simulink model "three_phase_pwm_rectifier_with_PMSGblock"  (R2015b)
settings: Solver=FixedStepAuto  SolverMode=SingleTasking  StartTime=0.0  StopTime=10.0  FixedStep=Ts  RelTol=1e-3
values from neighbouring files (symbols this model uses):
  Ts = 10e-6    (= 1e-05)    [three_phase_pwm_rectifier.m]
undefined symbols (not defined in the file or in its folder): fluxlinkage, gear, Jtotal, Ld, Lq, p, pgen, Prated, R, Rs, windspeed
libraries: powerlib x23, powerlib_meascontrol x9, simulink x7
settings Model: Creator=Eren  LastModifiedBy=Eren

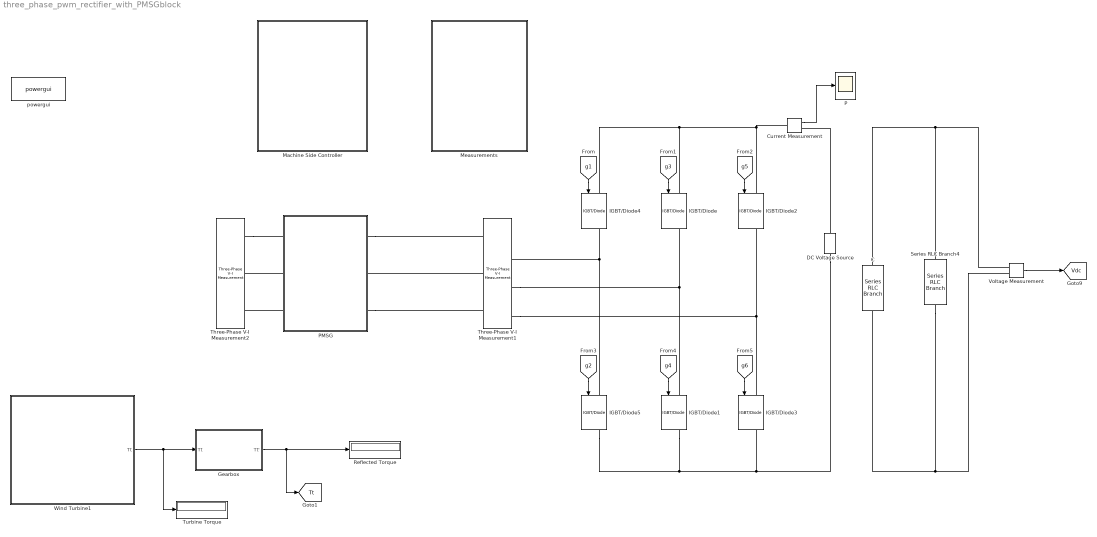
== system three_phase_pwm_rectifier_with_PMSGblock ==
  C : powerlib/Elements/Series RLC Branch  LConnTagsString=__new0  RConnTagsString=__new0  BranchType=C  Resistance=1  Inductance=1e-3  SetiL0=off  InitialCurrent=0  Capacitance=2700e-6  Setx0=on  InitialVoltage=1200  Measurements=None
  Current Measurement : powerlib/Measurements/Current Measurement  PhasorSimulation=off  OutputType=Complex  PSBequivalent=0
  DC Voltage Source : powerlib/Electrical Sources/DC Voltage Source  Amplitude=1200  Measurements=None
  Gearbox : Subsystem
  IGBT/Diode{,1..5} (6 alike) : powerlib/Power Electronics/IGBT//Diode  Ron=1e-3  Rs=1e5  Cs=inf  Measurements=on
  "Machine Side Controller " : Subsystem
  Measurements : Subsystem
  P : Scope
  "PMSG " : Subsystem
  Reflected Torque : Display
  Series RLC Branch4 : powerlib/Elements/Series RLC Branch  LConnTagsString=__new0  RConnTagsString=__new0  BranchType=R  Resistance=(1200)^2/2.75e6  Inductance=1e-3  SetiL0=off  InitialCurrent=0  Capacitance=1e-6  Setx0=off  InitialVoltage=0  Measurements=None
  Three-Phase V-I Measurement1 : powerlib/Measurements/Three-Phase V-I Measurement  VoltageMeasurement=phase-to-phase  SetLabelV=off  LabelV=Vsabc  Vpu=off  VpuLL=on  CurrentMeasurement=yes  SetLabelI=on  LabelI=Isabc  Ipu=on  Pbase=2.75e6  Vbase=690  OutputType=Complex  PhasorSimulation=off  PSBequivalent=0
  Three-Phase V-I Measurement2 : powerlib/Measurements/Three-Phase V-I Measurement  VoltageMeasurement=phase-to-phase  SetLabelV=on  LabelV=Vsabc  Vpu=off  VpuLL=on  CurrentMeasurement=no  SetLabelI=off  LabelI=Isabc  Ipu=off  Pbase=2.75e6  Vbase=690  OutputType=Complex  PhasorSimulation=off  PSBequivalent=0
  Turbine Torque : Display
  Voltage Measurement : powerlib/Measurements/Voltage Measurement  PhasorSimulation=off  OutputType=Complex  PSBequivalent=0
  Wind Turbine1 : Subsystem
  powergui : powerlib/powergui  Priority=2  SimulationMode=Discrete  SolverType=Tustin  SampleTime=Ts  frequency=60  SPID=off  DisableSnubberDevices=off  DisableRonSwitches=off  DisableVfSwitches=off  SwTol=0  DisplayEquations=off  Interpol=off  ExternalGateDelay=off  methode=off  Ts=0  FunctionMessages=off  echomessages=off  HookPort=off  EnableUseOfTLC=off  x0status=blocks  frequencyindice=0  Pbase=100e6  ErrMax=1e-4  Iterations=50  UnitsV=kV  UnitsW=MW  buscounter=0  RestoreLinks=warning  ResistiveCurrentMeasurement=off  Frange=[0:2:500]  Ylog=off  Xlog=on  ShowGrid=off  save=off  variable=ZData  structure=0  ZoomFFT=on  StartTime=0.0  cycles=1  DisplayStyle=1  fundamental=60  FreqAxis=off  MaxFrequency=1000  frequencyindicesteady=1  RmsSteady=1  display=off
  tag scope: Tt=global, Vdc=global
  wires:
  [g1] -> IGBT/Diode4/1
  [g3] -> IGBT/Diode/1
  [g5] -> IGBT/Diode2/1
  [g2] -> IGBT/Diode5/1
  [g4] -> IGBT/Diode1/1
  [g6] -> IGBT/Diode3/1
  Voltage Measurement/1 -> [Vdc]
  Current Measurement/1 -> P/1
  Wind Turbine1/1(Tt) -> Turbine Torque/1, Gearbox/1(Tt)
  Gearbox/1(Tt') -> [Tt], Reflected Torque/1
  connections:
  IGBT/Diode5/LConn1 -- IGBT/Diode4/RConn1 -- Three-Phase V-I Measurement1/RConn1
  IGBT/Diode1/LConn1 -- Three-Phase V-I Measurement1/RConn2 -- IGBT/Diode/RConn1
  IGBT/Diode3/LConn1 -- Three-Phase V-I Measurement1/RConn3 -- IGBT/Diode2/RConn1
  Series RLC Branch4/LConn1 -- Voltage Measurement/LConn1 -- C/LConn1
  IGBT/Diode2/LConn1 -- Current Measurement/LConn1 -- IGBT/Diode/LConn1 -- IGBT/Diode4/LConn1
  Voltage Measurement/LConn2 -- C/RConn1 -- Series RLC Branch4/RConn1
  "PMSG "/RConn1 -- Three-Phase V-I Measurement1/LConn1
  IGBT/Diode5/RConn1 -- IGBT/Diode3/RConn1 -- DC Voltage Source/LConn1 -- IGBT/Diode1/RConn1
  DC Voltage Source/RConn1 -- Current Measurement/RConn1
  "PMSG "/RConn3 -- Three-Phase V-I Measurement1/LConn3
  Three-Phase V-I Measurement1/LConn2 -- "PMSG "/RConn2
  Three-Phase V-I Measurement2/RConn1 -- "PMSG "/LConn1
  "PMSG "/LConn2 -- Three-Phase V-I Measurement2/RConn2
  "PMSG "/LConn3 -- Three-Phase V-I Measurement2/RConn3

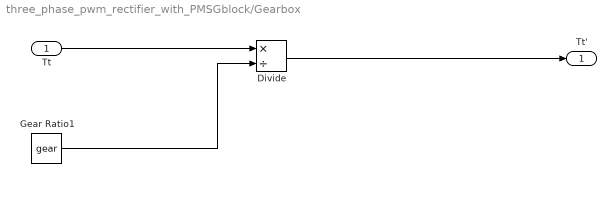
== system three_phase_pwm_rectifier_with_PMSGblock/Gearbox ==
  Tt : Inport
  Divide : Product  Inputs=*/
  Gear Ratio1 : Constant  Value=gear
  Tt' : Outport
  wires:
  Gear Ratio1/1 -> Divide/2
  Tt/1 -> Divide/1
  Divide/1 -> Tt'/1

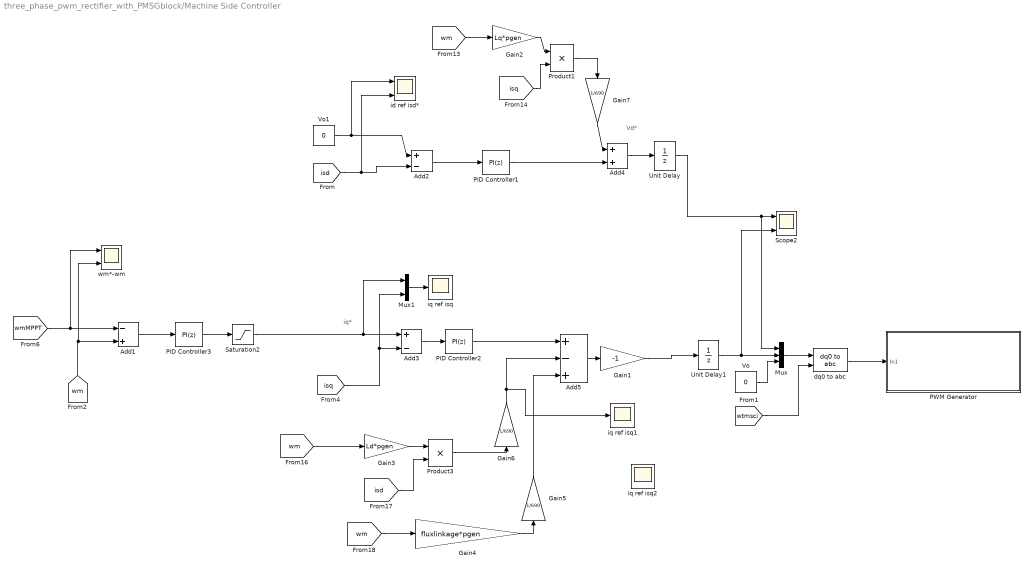
== system three_phase_pwm_rectifier_with_PMSGblock/Machine Side Controller  ==
  note: iq*
  note: Vd*
  Add1 : Sum  Inputs=-+
  Add2 : Sum  Inputs=+-
  Add3 : Sum  Inputs=+-
  Add4 : Sum
  Add5 : Sum  Inputs=+-+
  Gain1 : Gain  Gain=-1
  Gain2 : Gain  Gain=Lq*pgen
  Gain3 : Gain  Gain=Ld*pgen
  Gain4 : Gain  Gain=fluxlinkage*pgen
  Gain5 : Gain  Gain=1/690
  Gain6 : Gain  Gain=1/690
  Gain7 : Gain  Gain=1/690
  Mux : Mux  Inputs=3
  Mux1 : Mux  Inputs=2
  PID Controller1 : simulink/Continuous/PID Controller  Controller=PI  TimeDomain=Discrete-time  SampleTime=-1  IntegratorMethod=Forward Euler  FilterMethod=Forward Euler  Form=Ideal  UseFilter=on  ControllerParametersSource=internal  P=0.01  I=0.1  D=0  N=100  InitialConditionSource=internal  InitialConditionForIntegrator=0  InitialConditionForFilter=0  ExternalReset=none  LimitOutput=on  UpperSaturationLimit=1.5  LowerSaturationLimit=-1.5  LinearizeAsGain=on  AntiWindupMode=none  Kb=1  TrackingMode=off  Kt=1  PParamMin=[]  PParamMax=[]  IParamMin=[]  IParamMax=[]  DParamMin=[]  DParamMax=[]  NParamMin=[]  NParamMax=[]  KbParamMin=[]  KbParamMax=[]  KtParamMin=[]  KtParamMax=[]  POutMin=[]  POutMax=[]  IOutMin=[]  IOutMax=[]  DOutMin=[]  DOutMax=[]  NOutMin=[]  NOutMax=[]  KbOutMin=[]  KbOutMax=[]  KtOutMin=[]  KtOutMax=[]  IntegratorOutMin=[]  IntegratorOutMax=[]  FilterOutMin=[]  FilterOutMax=[]  SumOutMin=[]  SumOutMax=[]  SumI1OutMin=[]  SumI1OutMax=[]  SumI2OutMin=[]  SumI2OutMax=[]  SumI3OutMin=[]  SumI3OutMax=[]  SumDOutMin=[]  SumDOutMax=[]  SaturationOutMin=[]  SaturationOutMax=[]  IntegratorContinuousStateAttributes=''  IntegratorStateMustResolveToSignalObject=off  IntegratorRTWStateStorageClass=Auto  FilterContinuousStateAttributes=''  FilterStateMustResolveToSignalObject=off  FilterRTWStateStorageClass=Auto  DifferentiatorICPrevScaledInput=0  DifferentiatorOutMin=[]  DifferentiatorOutMax=[]
  PID Controller2 : simulink/Continuous/PID Controller  Controller=PI  TimeDomain=Discrete-time  SampleTime=-1  IntegratorMethod=Forward Euler  FilterMethod=Forward Euler  Form=Ideal  UseFilter=on  ControllerParametersSource=internal  P=0.1  I=1  D=0  N=100  InitialConditionSource=internal  InitialConditionForIntegrator=0  InitialConditionForFilter=0  ExternalReset=none  LimitOutput=on  UpperSaturationLimit=1.5  LowerSaturationLimit=-1.5  LinearizeAsGain=on  AntiWindupMode=none  Kb=1  TrackingMode=off  Kt=1  PParamMin=[]  PParamMax=[]  IParamMin=[]  IParamMax=[]  DParamMin=[]  DParamMax=[]  NParamMin=[]  NParamMax=[]  KbParamMin=[]  KbParamMax=[]  KtParamMin=[]  KtParamMax=[]  POutMin=[]  POutMax=[]  IOutMin=[]  IOutMax=[]  DOutMin=[]  DOutMax=[]  NOutMin=[]  NOutMax=[]  KbOutMin=[]  KbOutMax=[]  KtOutMin=[]  KtOutMax=[]  IntegratorOutMin=[]  IntegratorOutMax=[]  FilterOutMin=[]  FilterOutMax=[]  SumOutMin=[]  SumOutMax=[]  SumI1OutMin=[]  SumI1OutMax=[]  SumI2OutMin=[]  SumI2OutMax=[]  SumI3OutMin=[]  SumI3OutMax=[]  SumDOutMin=[]  SumDOutMax=[]  SaturationOutMin=[]  SaturationOutMax=[]  IntegratorContinuousStateAttributes=''  IntegratorStateMustResolveToSignalObject=off  IntegratorRTWStateStorageClass=Auto  FilterContinuousStateAttributes=''  FilterStateMustResolveToSignalObject=off  FilterRTWStateStorageClass=Auto  DifferentiatorICPrevScaledInput=0  DifferentiatorOutMin=[]  DifferentiatorOutMax=[]
  PID Controller3 : simulink/Continuous/PID Controller  Controller=PI  TimeDomain=Discrete-time  SampleTime=-1  IntegratorMethod=Forward Euler  FilterMethod=Forward Euler  Form=Ideal  UseFilter=on  ControllerParametersSource=internal  P=0.01  I=0.001  D=0  N=100  InitialConditionSource=internal  InitialConditionForIntegrator=0  InitialConditionForFilter=0  ExternalReset=none  LimitOutput=on  UpperSaturationLimit=1.5  LowerSaturationLimit=-1.5  LinearizeAsGain=on  AntiWindupMode=none  Kb=1  TrackingMode=off  Kt=1  PParamMin=[]  PParamMax=[]  IParamMin=[]  IParamMax=[]  DParamMin=[]  DParamMax=[]  NParamMin=[]  NParamMax=[]  KbParamMin=[]  KbParamMax=[]  KtParamMin=[]  KtParamMax=[]  POutMin=[]  POutMax=[]  IOutMin=[]  IOutMax=[]  DOutMin=[]  DOutMax=[]  NOutMin=[]  NOutMax=[]  KbOutMin=[]  KbOutMax=[]  KtOutMin=[]  KtOutMax=[]  IntegratorOutMin=[]  IntegratorOutMax=[]  FilterOutMin=[]  FilterOutMax=[]  SumOutMin=[]  SumOutMax=[]  SumI1OutMin=[]  SumI1OutMax=[]  SumI2OutMin=[]  SumI2OutMax=[]  SumI3OutMin=[]  SumI3OutMax=[]  SumDOutMin=[]  SumDOutMax=[]  SaturationOutMin=[]  SaturationOutMax=[]  IntegratorContinuousStateAttributes=''  IntegratorStateMustResolveToSignalObject=off  IntegratorRTWStateStorageClass=Auto  FilterContinuousStateAttributes=''  FilterStateMustResolveToSignalObject=off  FilterRTWStateStorageClass=Auto  DifferentiatorICPrevScaledInput=0  DifferentiatorOutMin=[]  DifferentiatorOutMax=[]
  "PWM Generator " : Subsystem
  Product1 : Product
  Product3 : Product
  Saturation2 : Saturate  UpperLimit=1.5  LowerLimit=0
  Scope2 : Scope  NumInputPorts=2
  Unit Delay : UnitDelay  SampleTime=Ts
  Unit Delay1 : UnitDelay  SampleTime=Ts
  Vo : Constant  Value=0
  Vo1 : Constant  Value=0
  dq0 to abc : powerlib_meascontrol/Transformations/dq0 to abc  Alignment=Aligned with phase A axis
  id ref isd* : Scope  NumInputPorts=2
  iq ref isq : Scope
  iq ref isq1 : Scope
  iq ref isq2 : Scope
  wm*-wm : Scope  NumInputPorts=2
  wires:
  Mux/1 -> dq0 to abc/1
  Vo1/1 -> id ref isd*/1, Add2/1
  Vo/1 -> Mux/3
  [isq] -> Add3/2, Mux1/2
  Add3/1 -> PID Controller2/1
  Add2/1 -> PID Controller1/1
  [isd] -> id ref isd*/2, Add2/2
  Mux1/1 -> iq ref isq/1
  [wtmsci] -> dq0 to abc/2
  [wm] -> wm*-wm/2, Add1/2
  [wmMPPT] -> wm*-wm/1, Add1/1
  Add1/1 -> PID Controller3/1
  dq0 to abc/1 -> "PWM Generator "/1(In1)
  Unit Delay/1 -> Mux/1, Scope2/1
  Unit Delay1/1 -> Mux/2, Scope2/2
  [wm] -> Gain2/1
  [isq] -> Product1/2
  Gain2/1 -> Product1/1
  Add4/1 -> Unit Delay/1
  PID Controller1/1 -> Add4/2
  Add5/1 -> Gain1/1
  PID Controller2/1 -> Add5/1
  [wm] -> Gain3/1
  Gain3/1 -> Product3/1
  [isd] -> Product3/2
  Product3/1 -> Gain6/1
  Gain4/1 -> Gain5/1
  [wm] -> Gain4/1
  Gain6/1 -> Add5/2, iq ref isq1/1
  Product1/1 -> Gain7/1
  Gain1/1 -> Unit Delay1/1
  PID Controller3/1 -> Saturation2/1
  Saturation2/1 -> Mux1/1, Add3/1
  Gain7/1 -> Add4/1
  Gain5/1 -> Add5/3

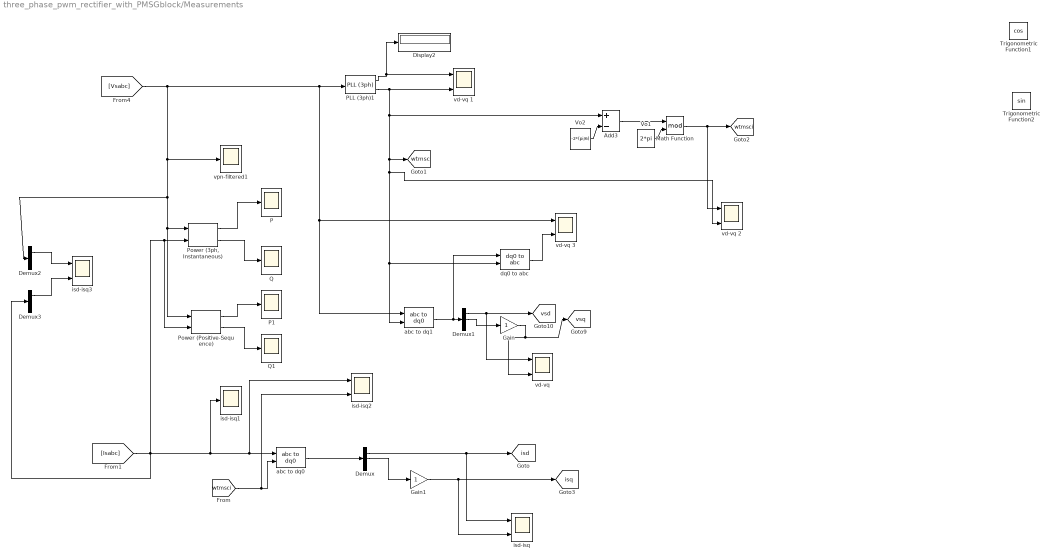
== system three_phase_pwm_rectifier_with_PMSGblock/Measurements ==
  Add3 : Sum  Inputs=+-
  Demux{,1..3} (4 alike) : Demux  Outputs=3
  Display2 : Display
  Gain : Gain
  Gain1 : Gain
  Math Function : Math  Operator=mod  SaturateOnIntegerOverflow=on
  P : Scope
  P1 : Scope
  PLL (3ph)1 : powerlib_meascontrol/PLL/PLL (3ph)  Fmin=55/3  Par_Init=[0, 50]  ParK=[180, 3200, 1]  TcD=1e-4  MaxRateChangeFreq=12  FilterCutOffFreq=25  Ts=0  AGC=on
  "Power (3ph, Instantaneous)" : powerlib_meascontrol/Measurements/Power (3ph, Instantaneous)
  Power (Positive-Sequence) : powerlib_meascontrol/Measurements/Power (Positive-Sequence)  Freq=60  Vinit=[0, 0]  Iinit=[0, 0]  Ts=0
  Q : Scope
  Q1 : Scope
  Trigonometric Function1 : Trigonometry  Operator=cos
  Trigonometric Function2 : Trigonometry
  Vo1 : Constant  Value=2*pi
  Vo2 : Constant  Value=-2*(pi/6)
  abc to dq0 : powerlib_meascontrol/Transformations/abc to dq0  Alignment=Aligned with phase A axis
  abc to dq1 : powerlib_meascontrol/Transformations/abc to dq0  Alignment=Aligned with phase A axis
  dq0 to abc : powerlib_meascontrol/Transformations/dq0 to abc  Alignment=Aligned with phase A axis
  isd-isq : Scope  NumInputPorts=2
  isd-isq1 : Scope
  isd-isq2 : Scope  NumInputPorts=2
  isd-isq3 : Scope  NumInputPorts=2
  vd-vq {,1..3} (4 alike) : Scope  NumInputPorts=2
  vpn-filtered1 : Scope
  tag scope: isd=global, isq=global, vsd=global, vsq=global, wtmsc=global, wtmsci=global
  wires:
  [Vsabc] -> Power (Positive-Sequence)/1, "Power (3ph, Instantaneous)"/1, Demux2/1, vpn-filtered1/1, PLL (3ph)1/1, vd-vq 3/1, abc to dq1/1
  PLL (3ph)1/1 -> Display2/1, vd-vq 1/1
  [Isabc] -> Power (Positive-Sequence)/2, "Power (3ph, Instantaneous)"/2, Demux3/1, isd-isq1/1, isd-isq2/1, abc to dq0/1
  abc to dq0/1 -> Demux/1
  abc to dq1/1 -> dq0 to abc/1, Demux1/1
  Demux1/1 -> "vd-vq "/1, [vsd]
  Demux1/2 -> Gain/1
  Demux/1 -> isd-isq/1, [isd]
  Demux/2 -> Gain1/1
  Math Function/1 -> vd-vq 2/1, [wtmsci]
  Add3/1 -> Math Function/1
  Vo2/1 -> Add3/2
  Vo1/1 -> Math Function/2
  [wtmsci] -> isd-isq2/2, abc to dq0/2
  PLL (3ph)1/2 -> Add3/1, [wtmsc], vd-vq 2/2, dq0 to abc/2, abc to dq1/2, vd-vq 1/2
  "Power (3ph, Instantaneous)"/1 -> P/1
  "Power (3ph, Instantaneous)"/2 -> Q/1
  Power (Positive-Sequence)/1 -> P1/1
  Power (Positive-Sequence)/2 -> Q1/1
  Gain/1 -> "vd-vq "/2, [vsq]
  Gain1/1 -> [isq], isd-isq/2
  dq0 to abc/1 -> vd-vq 3/2
  Demux2/1 -> isd-isq3/1
  Demux3/1 -> isd-isq3/2

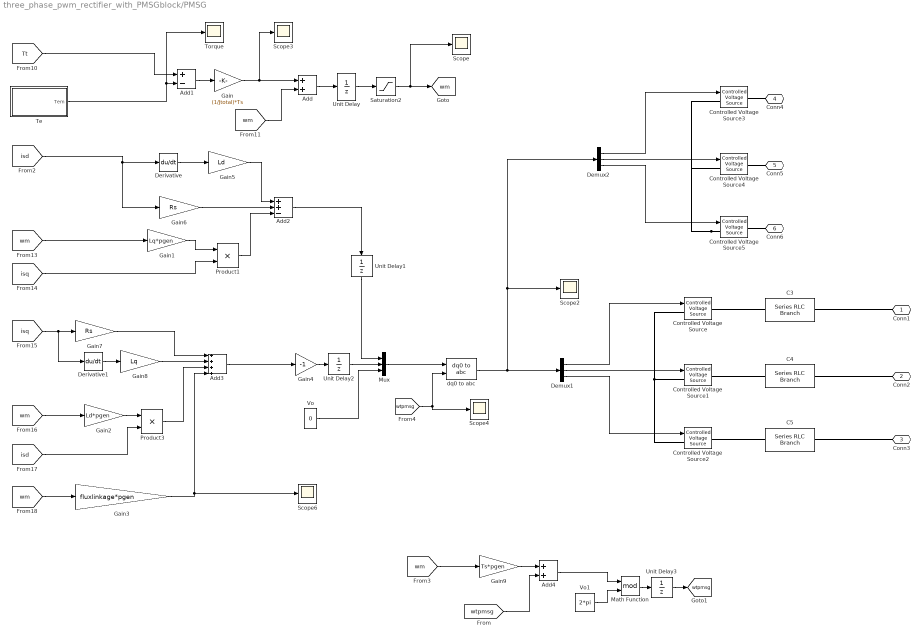
== system three_phase_pwm_rectifier_with_PMSGblock/PMSG  ==
  Add : Sum
  Add1 : Sum  Inputs=+-
  Add2 : Sum  Inputs=++-
  Add3 : Sum  Inputs=++++
  Add4 : Sum
  C3 : powerlib/Elements/Series RLC Branch  LConnTagsString=__new0  RConnTagsString=__new0  BranchType=RL  Resistance=Rs  Inductance=Lq  SetiL0=off  InitialCurrent=0  Capacitance=2700e-6  Setx0=on  InitialVoltage=1200  Measurements=None
  C4 : powerlib/Elements/Series RLC Branch  LConnTagsString=__new0  RConnTagsString=__new0  BranchType=RL  Resistance=Rs  Inductance=Lq  SetiL0=off  InitialCurrent=0  Capacitance=2700e-6  Setx0=on  InitialVoltage=1200  Measurements=None
  C5 : powerlib/Elements/Series RLC Branch  LConnTagsString=__new0  RConnTagsString=__new0  BranchType=RL  Resistance=Rs  Inductance=Lq  SetiL0=off  InitialCurrent=0  Capacitance=2700e-6  Setx0=on  InitialVoltage=1200  Measurements=None
  Controlled Voltage Source{,1..5} (6 alike) : powerlib/Electrical Sources/Controlled Voltage Source  Initialize=on  Source_Type=AC  Amplitude=0  Phase=0  Frequency=0  Measurements=None
  Demux1 : Demux  Outputs=3
  Demux2 : Demux  Outputs=3
  Derivative : Derivative
  Derivative1 : Derivative
  Gain : Gain  Gain=(1/Jtotal)*Ts
  Gain1 : Gain  Gain=Lq*pgen
  Gain2 : Gain  Gain=Ld*pgen
  Gain3 : Gain  Gain=fluxlinkage*pgen
  Gain4 : Gain  Gain=-1
  Gain5 : Gain  Gain=Ld
  Gain6 : Gain  Gain=Rs
  Gain7 : Gain  Gain=Rs
  Gain8 : Gain  Gain=Lq
  Gain9 : Gain  Gain=Ts*pgen
  Math Function : Math  Operator=mod  SaturateOnIntegerOverflow=on
  Mux : Mux  Inputs=3
  Product1 : Product
  Product3 : Product
  Saturation2 : Saturate  UpperLimit=2*pi*(1735/60)  LowerLimit=150
  Scope{,2..4,6} (5 alike) : Scope
  "Te " : Subsystem
  Torque : Scope
  Unit Delay : UnitDelay  SampleTime=Ts
  Unit Delay1 : UnitDelay  SampleTime=-1
  Unit Delay2 : UnitDelay  SampleTime=-1
  Unit Delay3 : UnitDelay  SampleTime=-1
  Vo : Constant  Value=0
  Vo1 : Constant  Value=2*pi
  dq0 to abc : powerlib_meascontrol/Transformations/dq0 to abc  Alignment=Aligned with phase A axis
  Conn1 : PMIOPort  Port=1  Side=Right
  Conn2 : PMIOPort  Port=2  Side=Right
  Conn3 : PMIOPort  Port=3  Side=Right
  Conn4 : PMIOPort  Port=4  Side=Left
  Conn5 : PMIOPort  Port=5  Side=Left
  Conn6 : PMIOPort  Port=6  Side=Left
  tag scope: wm=global, wtpmsg=global
  wires:
  Demux1/2 -> Controlled Voltage Source1/1
  Demux1/1 -> Controlled Voltage Source/1
  [wm] -> Gain1/1
  Add1/1 -> Gain/1
  Demux1/3 -> Controlled Voltage Source2/1
  [wm] -> Gain2/1
  Gain2/1 -> Product3/1
  [isd] -> Product3/2
  Gain7/1 -> Add3/1
  [isq] -> Derivative1/1, Gain7/1
  [wm] -> Add/2
  [isq] -> Product1/2
  Gain1/1 -> Product1/1
  Vo/1 -> Mux/3
  Mux/1 -> dq0 to abc/1
  Gain3/1 -> Add3/4, Scope6/1
  [wtpmsg] -> dq0 to abc/2, Scope4/1
  [wm] -> Gain3/1
  "Te "/1(Tem) -> Torque/1, Add1/2
  [Tt] -> Add1/1
  Gain/1 -> Scope3/1, Add/1
  Add/1 -> Unit Delay/1
  Unit Delay2/1 -> Mux/2
  Unit Delay1/1 -> Mux/1
  Add3/1 -> Gain4/1
  Gain4/1 -> Unit Delay2/1
  Demux2/2 -> Controlled Voltage Source4/1
  Demux2/1 -> Controlled Voltage Source3/1
  dq0 to abc/1 -> Scope2/1, Demux2/1, Demux1/1
  Demux2/3 -> Controlled Voltage Source5/1
  Unit Delay/1 -> Saturation2/1
  Saturation2/1 -> [wm], Scope/1
  Add2/1 -> Unit Delay1/1
  [isd] -> Gain6/1, Derivative/1
  Derivative/1 -> Gain5/1
  Product1/1 -> Add2/3
  Gain6/1 -> Add2/2
  Gain5/1 -> Add2/1
  Derivative1/1 -> Gain8/1
  Gain8/1 -> Add3/2
  Product3/1 -> Add3/3
  [wm] -> Gain9/1
  Gain9/1 -> Add4/1
  [wtpmsg] -> Add4/2
  Math Function/1 -> Unit Delay3/1
  Add4/1 -> Math Function/1
  Vo1/1 -> Math Function/2
  Unit Delay3/1 -> [wtpmsg]
  connections:
  Controlled Voltage Source/LConn1 -- Controlled Voltage Source1/LConn1 -- Controlled Voltage Source2/LConn1
  Controlled Voltage Source1/RConn1 -- C4/RConn1
  Controlled Voltage Source/RConn1 -- C3/RConn1
  C5/LConn1 -- Conn3/RConn1
  Controlled Voltage Source5/LConn1 -- Controlled Voltage Source3/LConn1 -- Controlled Voltage Source4/LConn1
  Controlled Voltage Source4/RConn1 -- Conn5/RConn1
  Controlled Voltage Source3/RConn1 -- Conn4/RConn1
  Controlled Voltage Source5/RConn1 -- Conn6/RConn1
  C3/LConn1 -- Conn1/RConn1
  C4/LConn1 -- Conn2/RConn1
  Controlled Voltage Source2/RConn1 -- C5/RConn1

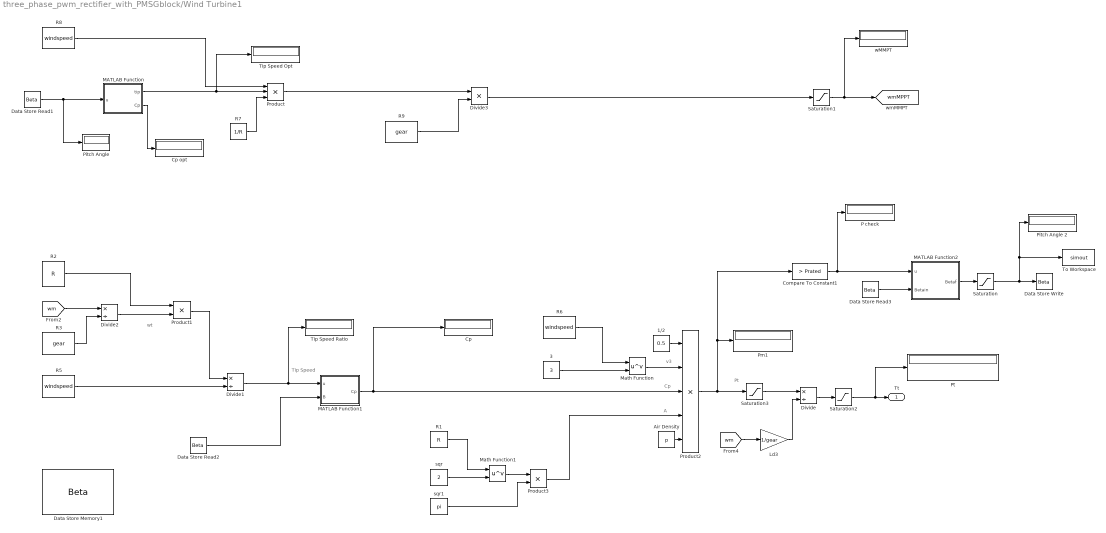
== system three_phase_pwm_rectifier_with_PMSGblock/Wind Turbine1 ==
  note: Pt
  note: v3
  note: Cp
  note: A
  note: wt
  note: Tip Speed
  1/2 : Constant  Value=0.5
  3 : Constant  Value=3
  Air Density : Constant  Value=p
  Compare To Constant1 : simulink/Logic and Bit Operations/Compare To Constant  relop=>  const=Prated  OutDataTypeStr=boolean
  Cp : Display
  Cp opt : Display
  Data Store Memory1 : DataStoreMemory  DataStoreName=Beta  ReadBeforeWriteMsg=warning  WriteAfterWriteMsg=warning  WriteAfterReadMsg=warning  OutMin=[0]  OutMax=[90]
  Data Store Read1 : DataStoreRead  DataStoreName=Beta  SampleTime=Ts
  Data Store Read2 : DataStoreRead  DataStoreName=Beta  SampleTime=Ts
  Data Store Read3 : DataStoreRead  DataStoreName=Beta  SampleTime=Ts
  Data Store Write : DataStoreWrite  DataStoreName=Beta
  Divide : Product  Inputs=*/
  Divide1 : Product  Inputs=*/
  Divide2 : Product  Inputs=*/
  Divide3 : Product  Inputs=**
  Ld3 : Gain  Gain=1/gear
  MATLAB Function : MATLAB Function  TreatAsAtomicUnit=on
  MATLAB Function1 : MATLAB Function  TreatAsAtomicUnit=on
  MATLAB Function2 : MATLAB Function  TreatAsAtomicUnit=on
  Math Function : Math  Operator=pow  SaturateOnIntegerOverflow=on
  Math Function1 : Math  Operator=pow  SaturateOnIntegerOverflow=on
  P check : Display
  "Pitch Angle " : Display
  Pitch Angle 2 : Display
  Pm1 : Display
  Product : Product  Inputs=3
  Product1 : Product
  Product2 : Product  Inputs=5
  Product3 : Product
  Pt : Display
  R1 : Constant  Value=R
  R2 : Constant  Value=R
  R3 : Constant  Value=gear
  R5 : Constant  Value=windspeed
  R6 : Constant  Value=windspeed
  R7 : Constant  Value=1/R
  R8 : Constant  Value=windspeed
  R9 : Constant  Value=gear
  Saturation : Saturate  UpperLimit=90  LowerLimit=0
  Saturation1 : Saturate  UpperLimit=181.68  LowerLimit=0
  Saturation2 : Saturate  UpperLimit=(2.75e6)/(2*pi*(550/60))*gear  LowerLimit=(2.75e6)/(2*pi*(1750/60))*gear
  Saturation3 : Saturate  UpperLimit=2.75e6  LowerLimit=0
  "Tip Speed Opt " : Display
  "Tip Speed Ratio " : Display
  To Workspace : ToWorkspace  VariableName=simout  SaveFormat=Timeseries  SampleTime=-1
  sqr : Constant  Value=2
  sqr1 : Constant  Value=pi
  "wMMPT " : Display
  Tt : Outport
  tag scope: wmMPPT=global
  wires:
  Air Density/1 -> Product2/5
  1/2/1 -> Product2/1
  Product3/1 -> Product2/4
  Math Function1/1 -> Product3/1
  sqr1/1 -> Product3/2
  [wm] -> Ld3/1
  Math Function/1 -> Product2/2
  sqr/1 -> Math Function1/2
  R1/1 -> Math Function1/1
  Product2/1 -> Saturation3/1, Compare To Constant1/1, Pm1/1
  3/1 -> Math Function/2
  R2/1 -> Product1/1
  [wm] -> Divide2/1
  Product1/1 -> Divide1/1
  R5/1 -> Divide1/2
  Divide1/1 -> MATLAB Function1/1(u), "Tip Speed Ratio "/1
  Divide2/1 -> Product1/2
  Ld3/1 -> Divide/2
  MATLAB Function1/1(Cp) -> Product2/3, Cp/1
  R3/1 -> Divide2/2
  R6/1 -> Math Function/1
  MATLAB Function/1(tip) -> "Tip Speed Opt "/1, Product/2
  R7/1 -> Product/3
  R8/1 -> Product/1
  Product/1 -> Divide3/1
  R9/1 -> Divide3/2
  MATLAB Function/2(Cp) -> Cp opt/1
  Divide3/1 -> Saturation1/1
  Data Store Read3/1 -> MATLAB Function2/2(Betain)
  Data Store Read2/1 -> MATLAB Function1/2(B)
  Data Store Read1/1 -> "Pitch Angle "/1, MATLAB Function/1(u)
  MATLAB Function2/1(Betaf) -> Saturation/1
  Compare To Constant1/1 -> MATLAB Function2/1(u), P check/1
  Saturation/1 -> To Workspace/1, Pitch Angle 2/1, Data Store Write/1
  Saturation1/1 -> "wMMPT "/1, [wmMPPT]
  Divide/1 -> Saturation2/1
  Saturation2/1 -> Pt/1, Tt/1
  Saturation3/1 -> Divide/1

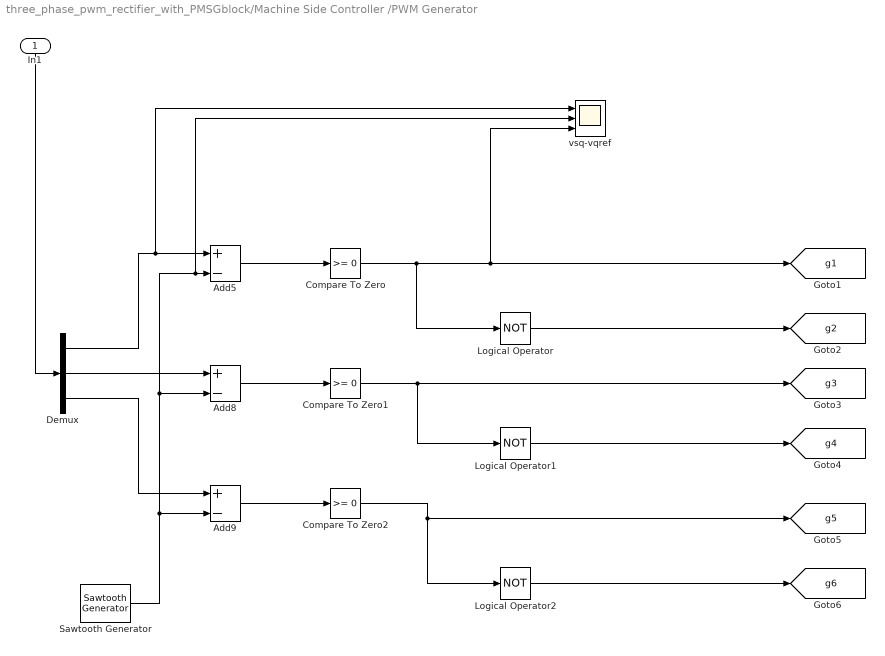
== system three_phase_pwm_rectifier_with_PMSGblock/Machine Side Controller /PWM Generator  ==
  In1 : Inport
  Add5 : Sum  Inputs=+-
  Add8 : Sum  Inputs=+-
  Add9 : Sum  Inputs=+-
  Compare To Zero : simulink/Logic and Bit Operations/Compare To Zero  relop=>=  OutDataTypeStr=boolean
  Compare To Zero1 : simulink/Logic and Bit Operations/Compare To Zero  relop=>=  OutDataTypeStr=boolean
  Compare To Zero2 : simulink/Logic and Bit Operations/Compare To Zero  relop=>=  OutDataTypeStr=boolean
  Demux : Demux  Outputs=3
  Logical Operator : Logic  Operator=NOT  AllPortsSameDT=off  OutDataTypeStr=boolean
  Logical Operator1 : Logic  Operator=NOT  AllPortsSameDT=off  OutDataTypeStr=boolean
  Logical Operator2 : Logic  Operator=NOT  AllPortsSameDT=off  OutDataTypeStr=boolean
  Sawtooth Generator : powerlib_meascontrol/Pulse & Signal Generators/Sawtooth Generator  Freq=drivefreq  Phase=0  Ts=Ts
  vsq-vqref : Scope  NumInputPorts=3
  tag scope: g1=global, g2=global, g3=global, g4=global, g5=global, g6=global
  wires:
  Add8/1 -> Compare To Zero1/1
  Demux/1 -> vsq-vqref/1, Add5/1
  Compare To Zero/1 -> Logical Operator/1, [g1], vsq-vqref/3
  Add9/1 -> Compare To Zero2/1
  Demux/2 -> Add8/1
  Demux/3 -> Add9/1
  Logical Operator2/1 -> [g6]
  Add5/1 -> Compare To Zero/1
  In1/1 -> Demux/1
  Sawtooth Generator/1 -> Add8/2, vsq-vqref/2, Add5/2, Add9/2
  Compare To Zero1/1 -> [g3], Logical Operator1/1
  Logical Operator/1 -> [g2]
  Compare To Zero2/1 -> Logical Operator2/1, [g5]
  Logical Operator1/1 -> [g4]

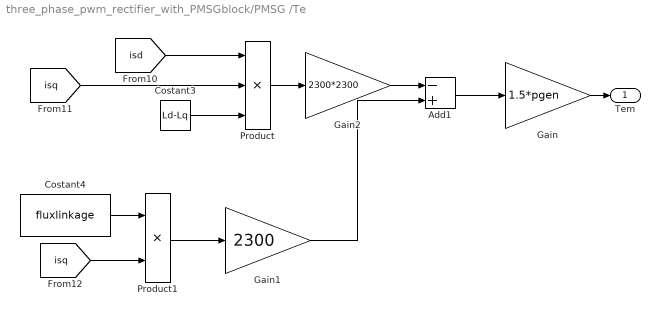
== system three_phase_pwm_rectifier_with_PMSGblock/PMSG /Te  ==
  Add1 : Sum  Inputs=-+
  Costant3 : Constant  Value=Ld-Lq
  Costant4 : Constant  Value=fluxlinkage
  Gain : Gain  Gain=1.5*pgen
  Gain1 : Gain  Gain=2300
  Gain2 : Gain  Gain=2300*2300
  Product : Product  Inputs=3
  Product1 : Product
  Tem : Outport
  wires:
  [isd] -> Product/1
  [isq] -> Product1/2
  Product1/1 -> Gain1/1
  Costant4/1 -> Product1/1
  Product/1 -> Gain2/1
  [isq] -> Product/2
  Costant3/1 -> Product/3
  Gain/1 -> Tem/1
  Add1/1 -> Gain/1
  Gain1/1 -> Add1/2
  Gain2/1 -> Add1/1

== matlab function three_phase_pwm_rectifier_with_PMSGblock/Wind Turbine1/MATLAB Function ==
  data: u input; tip output; Cp output
function [tip,Cp]= fcn(u)

c1 = 0.5176;
c2 = 116;
c3 = 0.4;
c4 = 5;
c5 = 21;
c6 = 0.0068;
B=0;
for i = 0.1:0.1:15
    
li = 1/((1/(i+0.08*u))-(0.035/(u^3+1)));
A = c1*((c2/li-c3*u-c4)*exp(-c5/li))+c6*i ;%#codegen

    if A < B
    lopt = i;
    break
    else 
    B = A;
    end
end
tip = i;
Cp = c1*((c2/li-c3*u-c4)*exp(-c5/li))+c6*i;
end

== matlab function three_phase_pwm_rectifier_with_PMSGblock/Wind Turbine1/MATLAB Function1 ==
  data: u input; B input; Cp output
function Cp = fcn(u,B)

c1 = 0.5176;
c2 = 116;
c3 = 0.4; 
c4 = 5;
c5 = 21;
c6 = 0.0068;

i =u;

li = 1/((1/(i+0.08*B))-(0.035/(B^3+1)));

Cp = c1*((c2/li-c3*B-c4)*exp(-c5/li))+c6*i;

end

== matlab function three_phase_pwm_rectifier_with_PMSGblock/Wind Turbine1/MATLAB Function2 ==
  data: u input; Betaf output; Betain input
function Betaf  = fcn(u,Betain)

    if u ==1
    Betaf = Betain+0.01;
    else  

    Betaf = Betain-0.01;
    end
 
    
    
end
